simulink model "Stochastic_Control"  (R2015b)
settings: Solver=VariableStepAuto  StartTime=0.0  StopTime=1000  RelTol=1e-3
settings Model: Creator=Jcama  LastModifiedBy=Jcama

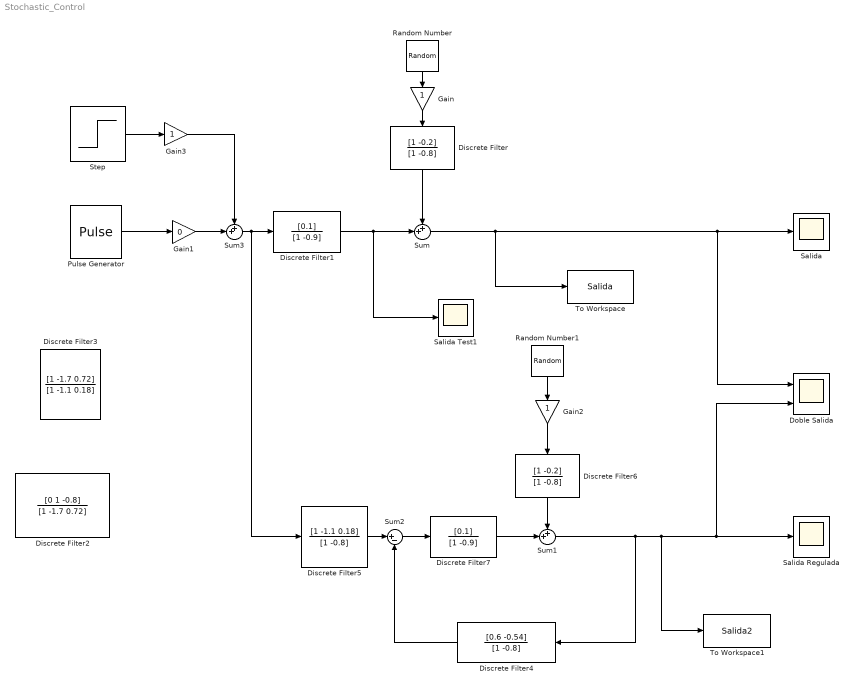
== system Stochastic_Control ==
  Discrete Filter : DiscreteFilter  Numerator=[1 -0.2]  Denominator=[1 -0.8]
  Discrete Filter1 : DiscreteFilter  Numerator=[0.1]  Denominator=[1 -0.9]
  Discrete Filter2 : DiscreteFilter  Numerator=[0 1 -0.8]  Denominator=[1 -1.7 0.72]
  Discrete Filter3 : DiscreteFilter  Numerator=[1 -1.7 0.72]  Denominator=[1 -1.1 0.18]
  Discrete Filter4 : DiscreteFilter  Numerator=[0.6 -0.54]  Denominator=[1 -0.8]
  Discrete Filter5 : DiscreteFilter  Numerator=[1 -1.1 0.18]  Denominator=[1 -0.8]
  Discrete Filter6 : DiscreteFilter  Numerator=[1 -0.2]  Denominator=[1 -0.8]
  Discrete Filter7 : DiscreteFilter  Numerator=[0.1]  Denominator=[1 -0.9]
  Doble Salida : Scope  NumInputPorts=2
  Gain : Gain
  Gain1 : Gain  Gain=0
  Gain2 : Gain
  Gain3 : Gain
  Pulse Generator : DiscretePulseGenerator  Amplitude=80  Period=200  PulseWidth=100  SampleTime=0.1
  Random Number : RandomNumber  Variance=0.6  SampleTime=0.1
  Random Number1 : RandomNumber  Variance=0.6  SampleTime=0.1
  Salida : Scope
  Salida Regulada : Scope
  Salida Test1 : Scope
  Step : Step  After=80  SampleTime=0.1
  Sum : Sum  Inputs=++|
  Sum1 : Sum  Inputs=++|
  Sum2 : Sum  Inputs=|+-
  Sum3 : Sum  Inputs=++|
  To Workspace : ToWorkspace  VariableName=Salida  SaveFormat=Timeseries  SampleTime=-1
  To Workspace1 : ToWorkspace  VariableName=Salida2  SaveFormat=Timeseries  SampleTime=-1
  wires:
  Gain/1 -> Discrete Filter/1
  Random Number/1 -> Gain/1
  Discrete Filter/1 -> Sum/1
  Discrete Filter1/1 -> Salida Test1/1, Sum/2
  Sum/1 -> To Workspace/1, Doble Salida/1, Salida/1
  Pulse Generator/1 -> Gain1/1
  Discrete Filter6/1 -> Sum1/1
  Gain2/1 -> Discrete Filter6/1
  Random Number1/1 -> Gain2/1
  Sum1/1 -> To Workspace1/1, Doble Salida/2, Salida Regulada/1, Discrete Filter4/1
  Discrete Filter4/1 -> Sum2/2
  Sum2/1 -> Discrete Filter7/1
  Discrete Filter5/1 -> Sum2/1
  Discrete Filter7/1 -> Sum1/2
  Step/1 -> Gain3/1
  Gain1/1 -> Sum3/2
  Gain3/1 -> Sum3/1
  Sum3/1 -> Discrete Filter5/1, Discrete Filter1/1
